simulink subsystem "INV_PWMsyncTask"  (R2022b)
settings: Solver=VariableStepAuto  StartTime=0.0  StopTime=10.0  RelTol=1e-3
values from neighbouring files (symbols this model uses):
  DPWM0Duclamp = [0 0 0 0 0 0 0 0 0 0 0 0 ... (1024 elements, 1024x1)]    [PWMLookUp.mat]    (also in prep_DPWM0_table.m = uint8(DPWM0Duclamp))
  DPWM0Dufi = [12288 12331 12374 12417 12458 12500 12541 12581 12621 12661 12700 12739 ... (1024 elements, 1024x1)]    [PWMLookUp.mat]    (also in prep_DPWM0_table.m = storedInteger(fixedPointValue))
  DPWM0Dusecfi = [-8192 -8192 -8192 -8192 -8192 -8192 -8192 -8192 -8192 -8192 -8192 -8192 ... (1024 elements, 1024x1)]    [PWMLookUp.mat]    (also in prep_DPWM0_table.m = storedInteger(fixedPointValue))
  DPWM0Dvclamp = [0 0 0 0 0 0 0 0 0 0 0 0 ... (1024 elements, 1024x1)]    [PWMLookUp.mat]    (also in prep_DPWM0_table.m = uint8(DPWM0Dvclamp))
  DPWM0Dvfi = [0 87 174 261 348 435 522 609 696 783 870 957 ... (1024 elements, 1024x1)]    [PWMLookUp.mat]    (also in prep_DPWM0_table.m = storedInteger(fixedPointValue))
  DPWM0Dvsecfi = [-8192 -8192 -8192 -8192 -8192 -8192 -8192 -8192 -8192 -8192 -8192 -8192 ... (1024 elements, 1024x1)]    [PWMLookUp.mat]    (also in prep_DPWM0_table.m = storedInteger(fixedPointValue))
  DPWM0Dwclamp = [2 2 2 2 2 2 2 2 2 2 2 2 ... (1024 elements, 1024x1)]    [PWMLookUp.mat]    (also in prep_DPWM0_table.m = uint8(DPWM0Dwclamp))
  DPWM0Dwfi = [0 0 0 0 0 0 0 0 0 0 0 0 ... (1024 elements, 1024x1)]    [PWMLookUp.mat]    (also in prep_DPWM0_table.m = storedInteger(fixedPointValue))
  DPWM0Dwsecfi = [-8192 -8192 -8192 -8192 -8192 -8192 -8192 -8192 -8192 -8192 -8192 -8192 ... (1024 elements, 1024x1)]    [PWMLookUp.mat]    (also in prep_DPWM0_table.m = storedInteger(fixedPointValue))
  DPWM1Duclamp = [1 1 1 1 1 1 1 1 1 1 1 1 ... (1024 elements, 1024x1)]    [PWMLookUp.mat]    (also in prep_DPWM1_table.m = uint8(DPWM1Duclamp))
  DPWM1Dufi = [0 0 0 0 0 0 0 0 0 0 0 0 ... (1024 elements, 1024x1)]    [PWMLookUp.mat]    (also in prep_DPWM1_table.m = storedInteger(fixedPointValue))
  DPWM1Dusecfi = [8192 8192 8192 8192 8192 8192 8192 8192 8192 8192 8192 8192 ... (1024 elements, 1024x1)]    [PWMLookUp.mat]    (also in prep_DPWM1_table.m = storedInteger(fixedPointValue))
  DPWM1Dvclamp = [0 0 0 0 0 0 0 0 0 0 0 0 ... (1024 elements, 1024x1)]    [PWMLookUp.mat]    (also in prep_DPWM1_table.m = uint8(DPWM1Dvclamp))
  DPWM1Dvfi = [-12288 -12244 -12200 -12155 -12110 -12065 -12019 -11972 -11925 -11878 -11830 -11782 ... (1024 elements, 1024x1)]    [PWMLookUp.mat]    (also in prep_DPWM1_table.m = storedInteger(fixedPointValue))
  DPWM1Dvsecfi = [8192 8192 8192 8192 8192 8192 8192 8192 8192 8192 8192 8192 ... (1024 elements, 1024x1)]    [PWMLookUp.mat]    (also in prep_DPWM1_table.m = storedInteger(fixedPointValue))
  DPWM1Dwclamp = [0 0 0 0 0 0 0 0 0 0 0 0 ... (1024 elements, 1024x1)]    [PWMLookUp.mat]    (also in prep_DPWM1_table.m = uint8(DPWM1Dwclamp))
  DPWM1Dwfi = [-12288 -12331 -12374 -12417 -12458 -12500 -12541 -12581 -12621 -12661 -12700 -12739 ... (1024 elements, 1024x1)]    [PWMLookUp.mat]    (also in prep_DPWM1_table.m = storedInteger(fixedPointValue))
  DPWM1Dwsecfi = [8192 8192 8192 8192 8192 8192 8192 8192 8192 8192 8192 8192 ... (1024 elements, 1024x1)]    [PWMLookUp.mat]    (also in prep_DPWM1_table.m = storedInteger(fixedPointValue))
  DPWM2Duclamp = [1 1 1 1 1 1 1 1 1 1 1 1 ... (1024 elements, 1024x1)]    [PWMLookUp.mat]    (also in prep_DPWM2_table.m = uint8(DPWM2Duclamp))
  DPWM2Dufi = [0 0 0 0 0 0 0 0 0 0 0 0 ... (1024 elements, 1024x1)]    [PWMLookUp.mat]    (also in prep_DPWM2_table.m = storedInteger(fixedPointValue))
  DPWM2Dusecfi = [8192 8192 8192 8192 8192 8192 8192 8192 8192 8192 8192 8192 ... (1024 elements, 1024x1)]    [PWMLookUp.mat]    (also in prep_DPWM2_table.m = storedInteger(fixedPointValue))
  DPWM2Dvclamp = [0 0 0 0 0 0 0 0 0 0 0 0 ... (1024 elements, 1024x1)]    [PWMLookUp.mat]    (also in prep_DPWM2_table.m = uint8(DPWM2Dvclamp))
  DPWM2Dvfi = [-12288 -12244 -12200 -12155 -12110 -12065 -12019 -11972 -11925 -11878 -11830 -11782 ... (1024 elements, 1024x1)]    [PWMLookUp.mat]    (also in prep_DPWM2_table.m = storedInteger(fixedPointValue))
  DPWM2Dvsecfi = [8192 8192 8192 8192 8192 8192 8192 8192 8192 8192 8192 8192 ... (1024 elements, 1024x1)]    [PWMLookUp.mat]    (also in prep_DPWM2_table.m = storedInteger(fixedPointValue))
  DPWM2Dwclamp = [0 0 0 0 0 0 0 0 0 0 0 0 ... (1024 elements, 1024x1)]    [PWMLookUp.mat]    (also in prep_DPWM2_table.m = uint8(DPWM2Dwclamp))
  DPWM2Dwfi = [-12288 -12331 -12374 -12417 -12458 -12500 -12541 -12581 -12621 -12661 -12700 -12739 ... (1024 elements, 1024x1)]    [PWMLookUp.mat]    (also in prep_DPWM2_table.m = storedInteger(fixedPointValue))
  DPWM2Dwsecfi = [8192 8192 8192 8192 8192 8192 8192 8192 8192 8192 8192 8192 ... (1024 elements, 1024x1)]    [PWMLookUp.mat]    (also in prep_DPWM2_table.m = storedInteger(fixedPointValue))
  DPWM3Duclamp = [0 0 0 0 0 0 0 0 0 0 0 0 ... (1024 elements, 1024x1)]    [PWMLookUp.mat]    (also in prep_DPWM3_table.m = uint8(DPWM3Duclamp))
  DPWM3Dufi = [12288 12331 12374 12417 12458 12500 12541 12581 12621 12661 12700 12739 ... (1024 elements, 1024x1)]    [PWMLookUp.mat]    (also in prep_DPWM3_table.m = storedInteger(fixedPointValue))
  DPWM3Dusecfi = [-8192 -8192 -8192 -8192 -8192 -8192 -8192 -8192 -8192 -8192 -8192 -8192 ... (1024 elements, 1024x1)]    [PWMLookUp.mat]    (also in prep_DPWM3_table.m = storedInteger(fixedPointValue))
  DPWM3Dvclamp = [0 0 0 0 0 0 0 0 0 0 0 0 ... (1024 elements, 1024x1)]    [PWMLookUp.mat]    (also in prep_DPWM3_table.m = uint8(DPWM3Dvclamp))
  DPWM3Dvfi = [0 87 174 261 348 435 522 609 696 783 870 957 ... (1024 elements, 1024x1)]    [PWMLookUp.mat]    (also in prep_DPWM3_table.m = storedInteger(fixedPointValue))
  DPWM3Dvsecfi = [-8192 -8192 -8192 -8192 -8192 -8192 -8192 -8192 -8192 -8192 -8192 -8192 ... (1024 elements, 1024x1)]    [PWMLookUp.mat]    (also in prep_DPWM3_table.m = storedInteger(fixedPointValue))
  DPWM3Dwclamp = [2 2 2 2 2 2 2 2 2 2 2 2 ... (1024 elements, 1024x1)]    [PWMLookUp.mat]    (also in prep_DPWM3_table.m = uint8(DPWM3Dwclamp))
  DPWM3Dwfi = [0 0 0 0 0 0 0 0 0 0 0 0 ... (1024 elements, 1024x1)]    [PWMLookUp.mat]    (also in prep_DPWM3_table.m = storedInteger(fixedPointValue))
  DPWM3Dwsecfi = [-8192 -8192 -8192 -8192 -8192 -8192 -8192 -8192 -8192 -8192 -8192 -8192 ... (1024 elements, 1024x1)]    [PWMLookUp.mat]    (also in prep_DPWM3_table.m = storedInteger(fixedPointValue))
  DPWMmaxDuclamp = [1 1 1 1 1 1 1 1 1 1 1 1 ... (1024 elements, 1024x1)]    [PWMLookUp.mat]    (also in prep_DPWMmax_table.m = uint8(DPWMmaxDuclamp))
  DPWMmaxDufi = [0 0 0 0 0 0 0 0 0 0 0 0 ... (1024 elements, 1024x1)]    [PWMLookUp.mat]    (also in prep_DPWMmax_table.m = storedInteger(fixedPointValue))
  DPWMmaxDusecfi = [8192 8192 8192 8192 8192 8192 8192 8192 8192 8192 8192 8192 ... (1024 elements, 1024x1)]    [PWMLookUp.mat]    (also in prep_DPWMmax_table.m = storedInteger(fixedPointValue))
  DPWMmaxDvclamp = [0 0 0 0 0 0 0 0 0 0 0 0 ... (1024 elements, 1024x1)]    [PWMLookUp.mat]    (also in prep_DPWMmax_table.m = uint8(DPWMmaxDvclamp))
  DPWMmaxDvfi = [-12288 -12244 -12200 -12155 -12110 -12065 -12019 -11972 -11925 -11878 -11830 -11782 ... (1024 elements, 1024x1)]    [PWMLookUp.mat]    (also in prep_DPWMmax_table.m = storedInteger(fixedPointValue))
  DPWMmaxDvsecfi = [8192 8192 8192 8192 8192 8192 8192 8192 8192 8192 8192 8192 ... (1024 elements, 1024x1)]    [PWMLookUp.mat]    (also in prep_DPWMmax_table.m = storedInteger(fixedPointValue))
  DPWMmaxDwclamp = [0 0 0 0 0 0 0 0 0 0 0 0 ... (1024 elements, 1024x1)]    [PWMLookUp.mat]    (also in prep_DPWMmax_table.m = uint8(DPWMmaxDwclamp))
  DPWMmaxDwfi = [-12288 -12331 -12374 -12417 -12458 -12500 -12541 -12581 -12621 -12661 -12700 -12739 ... (1024 elements, 1024x1)]    [PWMLookUp.mat]    (also in prep_DPWMmax_table.m = storedInteger(fixedPointValue))
  DPWMmaxDwsecfi = [8192 8192 8192 8192 8192 8192 8192 8192 8192 8192 8192 8192 ... (1024 elements, 1024x1)]    [PWMLookUp.mat]    (also in prep_DPWMmax_table.m = storedInteger(fixedPointValue))
  DPWMminDuclamp = [0 0 0 0 0 0 0 0 0 0 0 0 ... (1024 elements, 1024x1)]    [PWMLookUp.mat]    (also in prep_DPWMmin_table.m = uint8(DPWMminDuclamp))
  DPWMminDufi = [12288 12331 12374 12417 12458 12500 12541 12581 12621 12661 12700 12739 ... (1024 elements, 1024x1)]    [PWMLookUp.mat]    (also in prep_DPWMmin_table.m = storedInteger(fixedPointValue))
  DPWMminDusecfi = [-8192 -8192 -8192 -8192 -8192 -8192 -8192 -8192 -8192 -8192 -8192 -8192 ... (1024 elements, 1024x1)]    [PWMLookUp.mat]    (also in prep_DPWMmin_table.m = storedInteger(fixedPointValue))
  DPWMminDvclamp = [0 0 0 0 0 0 0 0 0 0 0 0 ... (1024 elements, 1024x1)]    [PWMLookUp.mat]    (also in prep_DPWMmin_table.m = uint8(DPWMminDvclamp))
  DPWMminDvfi = [0 87 174 261 348 435 522 609 696 783 870 957 ... (1024 elements, 1024x1)]    [PWMLookUp.mat]    (also in prep_DPWMmin_table.m = storedInteger(fixedPointValue))
  DPWMminDvsecfi = [-8192 -8192 -8192 -8192 -8192 -8192 -8192 -8192 -8192 -8192 -8192 -8192 ... (1024 elements, 1024x1)]    [PWMLookUp.mat]    (also in prep_DPWMmin_table.m = storedInteger(fixedPointValue))
  DPWMminDwclamp = [2 2 2 2 2 2 2 2 2 2 2 2 ... (1024 elements, 1024x1)]    [PWMLookUp.mat]    (also in prep_DPWMmin_table.m = uint8(DPWMminDwclamp))
  DPWMminDwfi = [0 0 0 0 0 0 0 0 0 0 0 0 ... (1024 elements, 1024x1)]    [PWMLookUp.mat]    (also in prep_DPWMmin_table.m = storedInteger(fixedPointValue))
  DPWMminDwsecfi = [-8192 -8192 -8192 -8192 -8192 -8192 -8192 -8192 -8192 -8192 -8192 -8192 ... (1024 elements, 1024x1)]    [PWMLookUp.mat]    (also in prep_DPWMmin_table.m = storedInteger(fixedPointValue))
  SPWMDufi = [8192 8192 8191 8191 8190 8188 8186 8184 8182 8180 8177 8173 ... (1024 elements, 1024x1)]    [PWMLookUp.mat]    (also in prep_SinePWM_table.m = storedInteger(fixedPointValue))
  SPWMDvfi = [-4096 -4052 -4009 -3965 -3921 -3876 -3832 -3788 -3743 -3698 -3653 -3608 ... (1024 elements, 1024x1)]    [PWMLookUp.mat]    (also in prep_SinePWM_table.m = storedInteger(fixedPointValue))
  SPWMDwfi = [-4096 -4139 -4183 -4226 -4269 -4312 -4354 -4397 -4439 -4481 -4523 -4565 ... (1024 elements, 1024x1)]    [PWMLookUp.mat]    (also in prep_SinePWM_table.m = storedInteger(fixedPointValue))
  SVPWMDufi = [6144 6166 6187 6208 6229 6250 6270 6291 6311 6330 6350 6369 ... (1024 elements, 1024x1)]    [PWMLookUp.mat]    (also in prep_SVPWM_table.m = storedInteger(fixedPointValue))
  SVPWMDvfi = [-6144 -6079 -6013 -5947 -5881 -5815 -5748 -5681 -5614 -5547 -5480 -5412 ... (1024 elements, 1024x1)]    [PWMLookUp.mat]    (also in prep_SVPWM_table.m = storedInteger(fixedPointValue))
  SVPWMDwfi = [-6144 -6166 -6187 -6208 -6229 -6250 -6270 -6291 -6311 -6330 -6350 -6369 ... (1024 elements, 1024x1)]    [PWMLookUp.mat]    (also in prep_SVPWM_table.m = storedInteger(fixedPointValue))
  THISPWMDufi = [6823 6823 6823 6823 6824 6825 6826 6827 6828 6829 6831 6832 ... (1024 elements, 1024x1)]    [PWMLookUp.mat]    (also in prep_THISPWM_table.m = storedInteger(fixedPointValue))
  THISPWMDvfi = [-5465 -5421 -5377 -5332 -5286 -5240 -5193 -5145 -5097 -5049 -4999 -4949 ... (1024 elements, 1024x1)]    [PWMLookUp.mat]    (also in prep_THISPWM_table.m = storedInteger(fixedPointValue))
  THISPWMDwfi = [-5465 -5508 -5551 -5593 -5634 -5675 -5715 -5755 -5794 -5832 -5869 -5906 ... (1024 elements, 1024x1)]    [PWMLookUp.mat]    (also in prep_THISPWM_table.m = storedInteger(fixedPointValue))
libraries: simulink x16
(part 2 of 2)

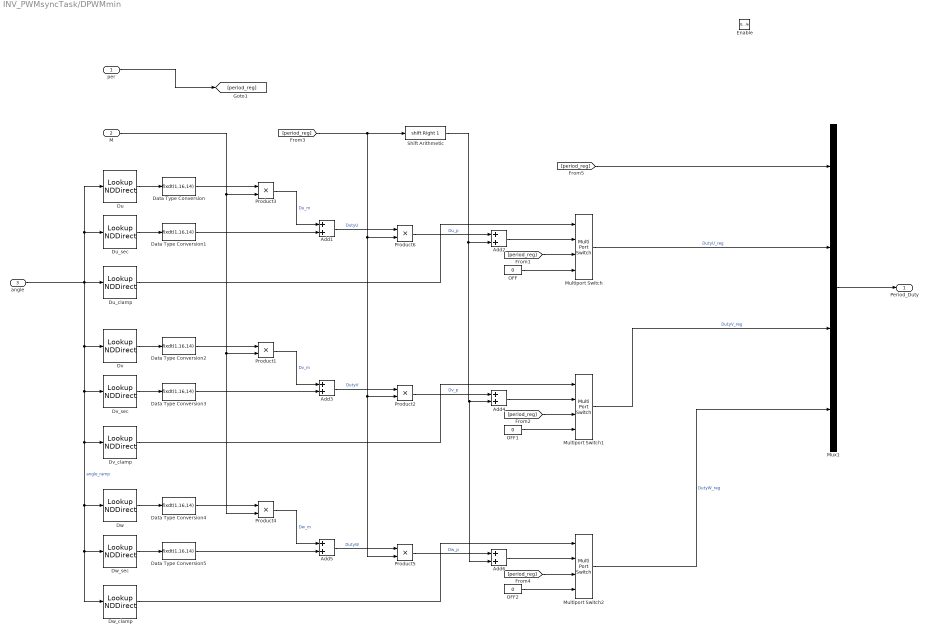
== system INV_PWMsyncTask/DPWMmin ==
  per : Inport
  M : Inport  Port=2
  angle : Inport  Port=3
  Enable : EnablePort
  Add1 : Sum  RndMeth=Simplest  OutDataTypeStr=Inherit: Same as first input
  Add2 : Sum  OutDataTypeStr=uint16  RndMeth=Simplest  SaturateOnIntegerOverflow=on
  Add3 : Sum  RndMeth=Simplest  OutDataTypeStr=Inherit: Same as first input
  Add4 : Sum  OutDataTypeStr=uint16  RndMeth=Simplest  SaturateOnIntegerOverflow=on
  Add5 : Sum  RndMeth=Simplest  OutDataTypeStr=Inherit: Same as first input
  Add6 : Sum  OutDataTypeStr=uint16  RndMeth=Simplest  SaturateOnIntegerOverflow=on
  Data Type Conversion{,1..5} (6 alike) : DataTypeConversion  OutDataTypeStr=fixdt(1,16,14)  ConvertRealWorld=Stored Integer (SI)  RndMeth=Simplest  SaturateOnIntegerOverflow=off
  Du : LookupNDDirect  NumberOfTableDimensions=1  Table=DPWMminDufi  DiagnosticForOutOfRangeInput=None  RemoveProtectionInput=on  TableDataTypeStr=int16
      settings: LockScale=on
  Du_clamp : LookupNDDirect  NumberOfTableDimensions=1  Table=DPWMminDuclamp  RemoveProtectionInput=on  TableDataTypeStr=uint8
      settings: LockScale=on
  Du_sec : LookupNDDirect  NumberOfTableDimensions=1  Table=DPWMminDusecfi  RemoveProtectionInput=on  TableDataTypeStr=int16
      settings: LockScale=on
  Dv : LookupNDDirect  NumberOfTableDimensions=1  Table=DPWMminDvfi  DiagnosticForOutOfRangeInput=None  RemoveProtectionInput=on  TableDataTypeStr=int16
      settings: LockScale=on
  Dv_clamp : LookupNDDirect  NumberOfTableDimensions=1  Table=DPWMminDvclamp  RemoveProtectionInput=on  TableDataTypeStr=uint8
      settings: LockScale=on
  Dv_sec : LookupNDDirect  NumberOfTableDimensions=1  Table=DPWMminDvsecfi  RemoveProtectionInput=on  TableDataTypeStr=int16
      settings: LockScale=on
  Dw : LookupNDDirect  NumberOfTableDimensions=1  Table=DPWMminDwfi  DiagnosticForOutOfRangeInput=None  RemoveProtectionInput=on  TableDataTypeStr=int16
      settings: LockScale=on
  Dw_clamp : LookupNDDirect  NumberOfTableDimensions=1  Table=DPWMminDwclamp  RemoveProtectionInput=on  TableDataTypeStr=uint8
      settings: LockScale=on
  Dw_sec : LookupNDDirect  NumberOfTableDimensions=1  Table=DPWMminDwsecfi  RemoveProtectionInput=on  TableDataTypeStr=int16
      settings: LockScale=on
  Multiport Switch : MultiPortSwitch  DataPortOrder=Zero-based contiguous  DiagnosticForDefault=None  zeroidx=on  SaturateOnIntegerOverflow=off  InputSameDT=off
  Multiport Switch1 : MultiPortSwitch  DataPortOrder=Zero-based contiguous  DiagnosticForDefault=None  zeroidx=on  SaturateOnIntegerOverflow=off  InputSameDT=off
  Multiport Switch2 : MultiPortSwitch  DataPortOrder=Zero-based contiguous  DiagnosticForDefault=None  zeroidx=on  SaturateOnIntegerOverflow=off  InputSameDT=off
  Mux1 : Mux
  OFF : Constant  Value=0  OutDataTypeStr=uint16  SampleTime=-1
  OFF1 : Constant  Value=0  OutDataTypeStr=uint16  SampleTime=-1
  OFF2 : Constant  Value=0  OutDataTypeStr=uint16  SampleTime=-1
  Product1 : Product  RndMeth=Simplest  OutDataTypeStr=Inherit: Same as first input  LockScale=on
  Product2 : Product  OutDataTypeStr=int16  RndMeth=Simplest
  Product3 : Product  RndMeth=Simplest  OutDataTypeStr=Inherit: Same as first input  LockScale=on
  Product4 : Product  RndMeth=Simplest  OutDataTypeStr=Inherit: Same as first input  LockScale=on
  Product5 : Product  OutDataTypeStr=int16  RndMeth=Simplest
  Product6 : Product  OutDataTypeStr=int16  RndMeth=Simplest
  Shift Arithmetic : ArithShift  BitShiftNumber=1  BitShiftDirection=Right
  Period_Duty : Outport
  wires:
  [period_reg] -> Mux1/1
  Multiport Switch/1 -> Mux1/2  "DutyU_reg"
  Multiport Switch1/1 -> Mux1/3  "DutyV_reg"
  Multiport Switch2/1 -> Mux1/4  "DutyW_reg"
  Mux1/1 -> Period_Duty/1
  per/1 -> [period_reg]
  Add2/1 -> Multiport Switch/2
  Data Type Conversion/1 -> Product3/1
  Product6/1 -> Add2/1  "Du_p"
  Du/1 -> Data Type Conversion/1
  Product3/1 -> Add1/1  "Du_m"
  Du_sec/1 -> Data Type Conversion1/1
  Add1/1 -> Product6/1  "DutyU"
  [period_reg] -> Multiport Switch/3
  OFF/1 -> Multiport Switch/4
  Du_clamp/1 -> Multiport Switch/1
  Data Type Conversion1/1 -> Add1/2
  Dv_clamp/1 -> Multiport Switch1/1
  Product1/1 -> Add3/1  "Dv_m"
  OFF1/1 -> Multiport Switch1/4
  Data Type Conversion3/1 -> Add3/2
  Add4/1 -> Multiport Switch1/2
  Data Type Conversion2/1 -> Product1/1
  Add3/1 -> Product2/1  "DutyV"
  [period_reg] -> Multiport Switch1/3
  Dv/1 -> Data Type Conversion2/1
  Dv_sec/1 -> Data Type Conversion3/1
  Product2/1 -> Add4/1  "Dv_p"
  [period_reg] -> Shift Arithmetic/1, Product5/2, Product2/2, Product6/2
  Dw_sec/1 -> Data Type Conversion5/1
  M/1 -> Product4/2, Product1/2, Product3/2
  Shift Arithmetic/1 -> Add2/2, Add6/2, Add4/2
  angle/1 -> Dv_clamp/1, Dw_clamp/1, Dw_sec/1, Dw/1, Dv_sec/1, Dv/1, Du_sec/1, Du/1, Du_clamp/1  "angle_ramp"
  [period_reg] -> Multiport Switch2/3
  Data Type Conversion5/1 -> Add5/2
  Add6/1 -> Multiport Switch2/2
  Add5/1 -> Product5/1  "DutyW"
  Dw/1 -> Data Type Conversion4/1
  Dw_clamp/1 -> Multiport Switch2/1
  OFF2/1 -> Multiport Switch2/4
  Product4/1 -> Add5/1  "Dw_m"
  Data Type Conversion4/1 -> Product4/1
  Product5/1 -> Add6/1  "Dw_p"

== system INV_PWMsyncTask/NORMAL_PWM ==
  Period_Duty_IN : Inport
  Action Port : ActionPort
  Period_Duty_OUT : Outport
  wires:
  Period_Duty_IN/1 -> Period_Duty_OUT/1

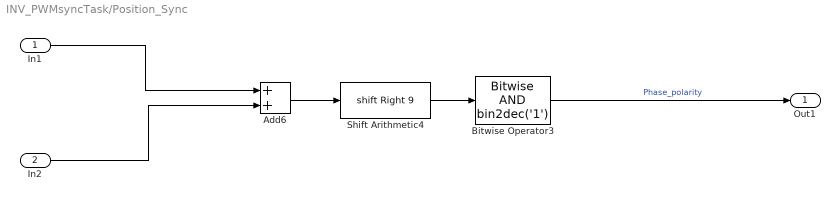
== system INV_PWMsyncTask/Position_Sync ==
  In1 : Inport
  In2 : Inport  Port=2
  Add6 : Sum
  Bitwise Operator3 : simulink/Logic and Bit Operations/Bitwise Operator  logicop=AND  UseBitMask=on  BitMask=bin2dec('1')  BitMaskRealWorld=Stored Integer
  Shift Arithmetic4 : ArithShift  BitShiftNumber=9  BitShiftDirection=Right
  Out1 : Outport
  wires:
  Add6/1 -> Shift Arithmetic4/1
  Bitwise Operator3/1 -> Out1/1  "Phase_polarity"
  In1/1 -> Add6/1
  Shift Arithmetic4/1 -> Bitwise Operator3/1
  In2/1 -> Add6/2

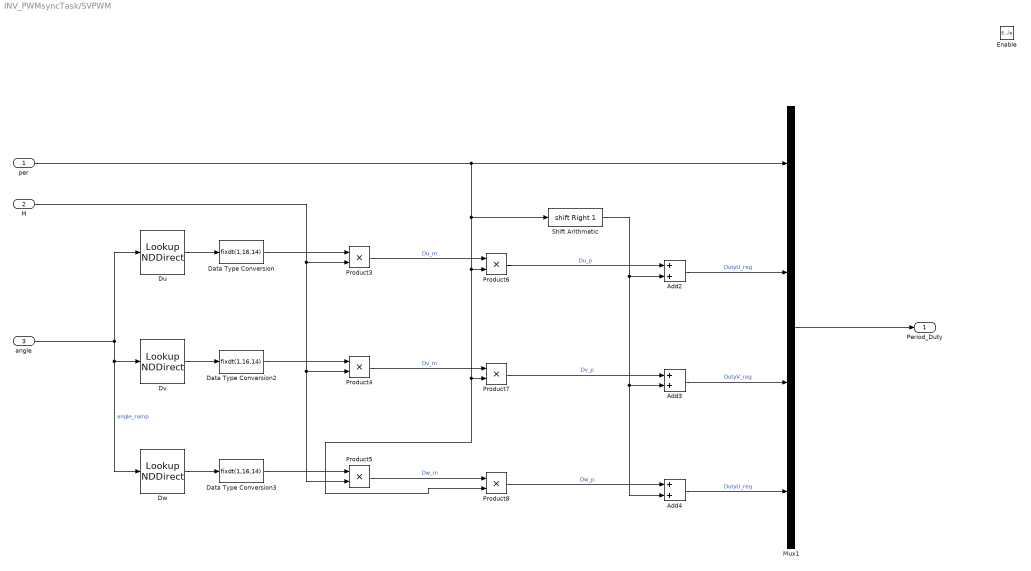
== system INV_PWMsyncTask/SVPWM ==
  per : Inport
  M : Inport  Port=2
  angle : Inport  Port=3
  Enable : EnablePort
  Add2 : Sum  OutDataTypeStr=uint16  RndMeth=Simplest  SaturateOnIntegerOverflow=on
  Add3 : Sum  OutDataTypeStr=uint16  RndMeth=Simplest  SaturateOnIntegerOverflow=on
  Add4 : Sum  OutDataTypeStr=uint16  RndMeth=Simplest  SaturateOnIntegerOverflow=on
  Data Type Conversion : DataTypeConversion  OutDataTypeStr=fixdt(1,16,14)  ConvertRealWorld=Stored Integer (SI)  SaturateOnIntegerOverflow=off  RndMeth=Floor
  Data Type Conversion2 : DataTypeConversion  OutDataTypeStr=fixdt(1,16,14)  ConvertRealWorld=Stored Integer (SI)  SaturateOnIntegerOverflow=off  RndMeth=Floor
  Data Type Conversion3 : DataTypeConversion  OutDataTypeStr=fixdt(1,16,14)  ConvertRealWorld=Stored Integer (SI)  SaturateOnIntegerOverflow=off  RndMeth=Floor
  Du : LookupNDDirect  NumberOfTableDimensions=1  Table=SVPWMDufi  RemoveProtectionInput=on  TableDataTypeStr=int16
      settings: LockScale=on
  Dv : LookupNDDirect  NumberOfTableDimensions=1  Table=SVPWMDvfi  DiagnosticForOutOfRangeInput=None  RemoveProtectionInput=on  TableDataTypeStr=int16
      settings: LockScale=on
  Dw : LookupNDDirect  NumberOfTableDimensions=1  Table=SVPWMDwfi  DiagnosticForOutOfRangeInput=None  RemoveProtectionInput=on  TableDataTypeStr=int16
      settings: LockScale=on
  Mux1 : Mux
  Product3 : Product  OutDataTypeStr=fixdt(1,16,14)  RndMeth=Simplest  LockScale=on
  Product4 : Product  OutDataTypeStr=fixdt(1,16,14)  RndMeth=Simplest  LockScale=on
  Product5 : Product  OutDataTypeStr=fixdt(1,16,14)  RndMeth=Simplest  LockScale=on
  Product6 : Product  OutDataTypeStr=int16  RndMeth=Simplest
  Product7 : Product  OutDataTypeStr=int16  RndMeth=Simplest
  Product8 : Product  OutDataTypeStr=int16  RndMeth=Simplest
  Shift Arithmetic : ArithShift  BitShiftNumber=1  BitShiftDirection=Right
  Period_Duty : Outport
  wires:
  Mux1/1 -> Period_Duty/1
  Product4/1 -> Product7/1  "Dv_m"
  M/1 -> Product5/2, Product4/2, Product3/2
  Add2/1 -> Mux1/2  "DutyU_reg"
  Product8/1 -> Add4/1  "Dw_p"
  Data Type Conversion/1 -> Product3/1
  Product6/1 -> Add2/1  "Du_p"
  Du/1 -> Data Type Conversion/1
  per/1 -> Mux1/1, Product8/2, Product7/2, Product6/2, Shift Arithmetic/1
  Product3/1 -> Product6/1  "Du_m"
  Shift Arithmetic/1 -> Add4/2, Add3/2, Add2/2
  Dw/1 -> Data Type Conversion3/1
  Add3/1 -> Mux1/3  "DutyV_reg"
  Product5/1 -> Product8/1  "Dw_m"
  Data Type Conversion3/1 -> Product5/1
  Data Type Conversion2/1 -> Product4/1
  Dv/1 -> Data Type Conversion2/1
  Add4/1 -> Mux1/4  "DutyU_reg"
  angle/1 -> Dw/1, Dv/1, Du/1  "angle_ramp"
  Product7/1 -> Add3/1  "Dv_p"

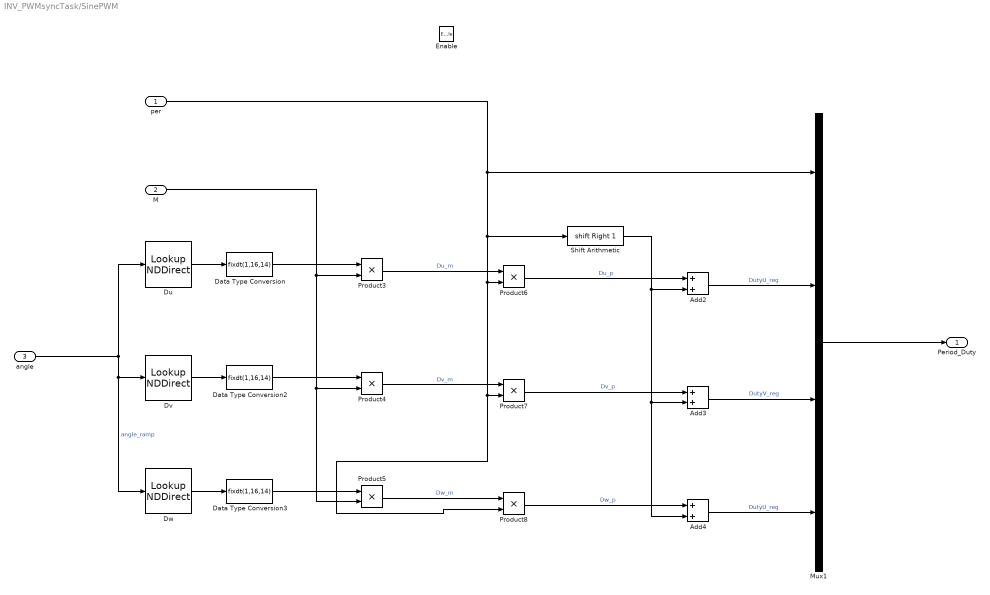
== system INV_PWMsyncTask/SinePWM ==
  per : Inport
  M : Inport  Port=2
  angle : Inport  Port=3
  Enable : EnablePort
  Add2 : Sum  OutDataTypeStr=uint16  RndMeth=Simplest  SaturateOnIntegerOverflow=on
  Add3 : Sum  OutDataTypeStr=uint16  RndMeth=Simplest  SaturateOnIntegerOverflow=on
  Add4 : Sum  OutDataTypeStr=uint16  RndMeth=Simplest  SaturateOnIntegerOverflow=on
  Data Type Conversion : DataTypeConversion  OutDataTypeStr=fixdt(1,16,14)  ConvertRealWorld=Stored Integer (SI)  SaturateOnIntegerOverflow=off  RndMeth=Floor
  Data Type Conversion2 : DataTypeConversion  OutDataTypeStr=fixdt(1,16,14)  ConvertRealWorld=Stored Integer (SI)  SaturateOnIntegerOverflow=off  RndMeth=Floor
  Data Type Conversion3 : DataTypeConversion  OutDataTypeStr=fixdt(1,16,14)  ConvertRealWorld=Stored Integer (SI)  SaturateOnIntegerOverflow=off  RndMeth=Floor
  Du : LookupNDDirect  NumberOfTableDimensions=1  Table=SPWMDufi  RemoveProtectionInput=on  TableDataTypeStr=int16
      settings: LockScale=on
  Dv : LookupNDDirect  NumberOfTableDimensions=1  Table=SPWMDvfi  DiagnosticForOutOfRangeInput=None  RemoveProtectionInput=on  TableDataTypeStr=int16
      settings: LockScale=on
  Dw : LookupNDDirect  NumberOfTableDimensions=1  Table=SPWMDwfi  DiagnosticForOutOfRangeInput=None  RemoveProtectionInput=on  TableDataTypeStr=int16
      settings: LockScale=on
  Mux1 : Mux
  Product3 : Product  OutDataTypeStr=fixdt(1,16,14)  RndMeth=Simplest  LockScale=on
  Product4 : Product  OutDataTypeStr=fixdt(1,16,14)  RndMeth=Simplest  LockScale=on
  Product5 : Product  OutDataTypeStr=fixdt(1,16,14)  RndMeth=Simplest  LockScale=on
  Product6 : Product  OutDataTypeStr=int16  RndMeth=Simplest
  Product7 : Product  OutDataTypeStr=int16  RndMeth=Simplest
  Product8 : Product  OutDataTypeStr=int16  RndMeth=Simplest
  Shift Arithmetic : ArithShift  BitShiftNumber=1  BitShiftDirection=Right
  Period_Duty : Outport
  wires:
  per/1 -> Product8/2, Product7/2, Product6/2, Shift Arithmetic/1, Mux1/1
  Mux1/1 -> Period_Duty/1
  Add4/1 -> Mux1/4  "DutyU_reg"
  Add3/1 -> Mux1/3  "DutyV_reg"
  Add2/1 -> Mux1/2  "DutyU_reg"
  Product4/1 -> Product7/1  "Dv_m"
  M/1 -> Product5/2, Product4/2, Product3/2
  Product8/1 -> Add4/1  "Dw_p"
  Data Type Conversion/1 -> Product3/1
  Product6/1 -> Add2/1  "Du_p"
  Du/1 -> Data Type Conversion/1
  Product3/1 -> Product6/1  "Du_m"
  Shift Arithmetic/1 -> Add4/2, Add3/2, Add2/2
  Dw/1 -> Data Type Conversion3/1
  Product5/1 -> Product8/1  "Dw_m"
  Data Type Conversion3/1 -> Product5/1
  Data Type Conversion2/1 -> Product4/1
  Dv/1 -> Data Type Conversion2/1
  angle/1 -> Dw/1, Dv/1, Du/1  "angle_ramp"
  Product7/1 -> Add3/1  "Dv_p"

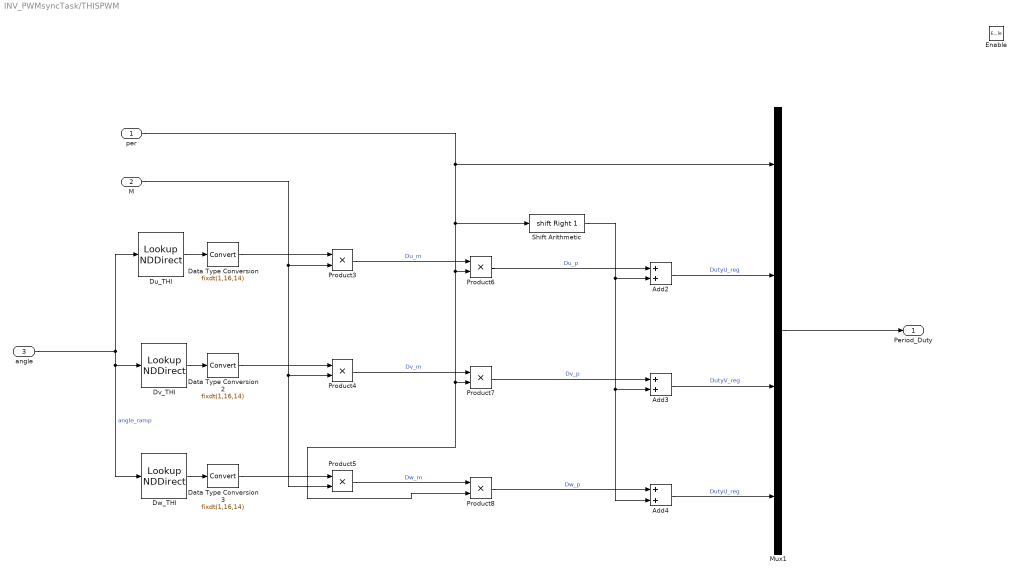
== system INV_PWMsyncTask/THISPWM ==
  per : Inport
  M : Inport  Port=2
  angle : Inport  Port=3
  Enable : EnablePort
  Add2 : Sum  OutDataTypeStr=uint16  RndMeth=Simplest  SaturateOnIntegerOverflow=on
  Add3 : Sum  OutDataTypeStr=uint16  RndMeth=Simplest  SaturateOnIntegerOverflow=on
  Add4 : Sum  OutDataTypeStr=uint16  RndMeth=Simplest  SaturateOnIntegerOverflow=on
  Data Type Conversion : DataTypeConversion  OutDataTypeStr=fixdt(1,16,14)  ConvertRealWorld=Stored Integer (SI)  SaturateOnIntegerOverflow=off  RndMeth=Floor
  Data Type Conversion2 : DataTypeConversion  OutDataTypeStr=fixdt(1,16,14)  ConvertRealWorld=Stored Integer (SI)  SaturateOnIntegerOverflow=off  RndMeth=Floor
  Data Type Conversion3 : DataTypeConversion  OutDataTypeStr=fixdt(1,16,14)  ConvertRealWorld=Stored Integer (SI)  SaturateOnIntegerOverflow=off  RndMeth=Floor
  Du_THI : LookupNDDirect  NumberOfTableDimensions=1  Table=THISPWMDufi  RemoveProtectionInput=on  TableDataTypeStr=int16
      settings: LockScale=on
  Dv_THI : LookupNDDirect  NumberOfTableDimensions=1  Table=THISPWMDvfi  DiagnosticForOutOfRangeInput=None  RemoveProtectionInput=on  TableDataTypeStr=int16
      settings: LockScale=on
  Dw_THI : LookupNDDirect  NumberOfTableDimensions=1  Table=THISPWMDwfi  DiagnosticForOutOfRangeInput=None  RemoveProtectionInput=on  TableDataTypeStr=int16
      settings: LockScale=on
  Mux1 : Mux
  Product3 : Product  OutDataTypeStr=fixdt(1,16,14)  RndMeth=Simplest  LockScale=on
  Product4 : Product  OutDataTypeStr=fixdt(1,16,14)  RndMeth=Simplest  LockScale=on
  Product5 : Product  OutDataTypeStr=fixdt(1,16,14)  RndMeth=Simplest  LockScale=on
  Product6 : Product  OutDataTypeStr=int16  RndMeth=Simplest
  Product7 : Product  OutDataTypeStr=int16  RndMeth=Simplest
  Product8 : Product  OutDataTypeStr=int16  RndMeth=Simplest
  Shift Arithmetic : ArithShift  BitShiftNumber=1  BitShiftDirection=Right
  Period_Duty : Outport
  wires:
  per/1 -> Product8/2, Product7/2, Product6/2, Shift Arithmetic/1, Mux1/1
  Mux1/1 -> Period_Duty/1
  Add4/1 -> Mux1/4  "DutyU_reg"
  Add3/1 -> Mux1/3  "DutyV_reg"
  Add2/1 -> Mux1/2  "DutyU_reg"
  Product4/1 -> Product7/1  "Dv_m"
  M/1 -> Product5/2, Product4/2, Product3/2
  Product8/1 -> Add4/1  "Dw_p"
  Data Type Conversion/1 -> Product3/1
  Product6/1 -> Add2/1  "Du_p"
  Du_THI/1 -> Data Type Conversion/1
  Product3/1 -> Product6/1  "Du_m"
  Shift Arithmetic/1 -> Add4/2, Add3/2, Add2/2
  Dw_THI/1 -> Data Type Conversion3/1
  Product5/1 -> Product8/1  "Dw_m"
  Data Type Conversion3/1 -> Product5/1
  Data Type Conversion2/1 -> Product4/1
  Dv_THI/1 -> Data Type Conversion2/1
  angle/1 -> Dv_THI/1, Dw_THI/1, Du_THI/1  "angle_ramp"
  Product7/1 -> Add3/1  "Dv_p"
